simulink model "dynamics"  (R2016b)
settings: Solver=VariableStepAuto  StartTime=0.0  StopTime=10.0  RelTol=1e-3
values from neighbouring files (symbols this model uses):
  ModelInit_RPM = 557.1420    (= 557.142)    [Init.m]
  ModelParam_envGravityAcc = 9.8    [Init.m]
  ModelParam_motorCr = 1148*2    (= 2296)    [Init.m]
  ModelParam_motorJm = 0.0001287    [Init.m]
  ModelParam_motorT = 0.02    [Init.m]
  ModelParam_motorWb = -141.4    [Init.m]
  ModelParam_rotorCm = 1.779e-07    [Init.m]
  ModelParam_rotorCt = 1.105e-05    [Init.m]
  ModelParam_uavCd = 0.073    [Init.m]
  ModelParam_uavJ = [ModelParam_uavJxx,0,0;0,ModelParam_uavJyy,0;0,0,ModelParam_uavJzz]    [Init.m]
  ModelParam_uavMass = 1.4    [Init.m]
  ModelParam_uavR = 0.225    [Init.m]
libraries: aerolibutil x2, aerolibtransform2 x2
settings Model: Creator=Mr Wang  LastModifiedBy=Mr Wang

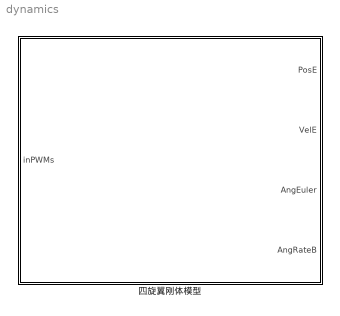
== system dynamics ==
  四旋翼刚体模型 : Subsystem
      mask Display: image('./icon/F450.png');

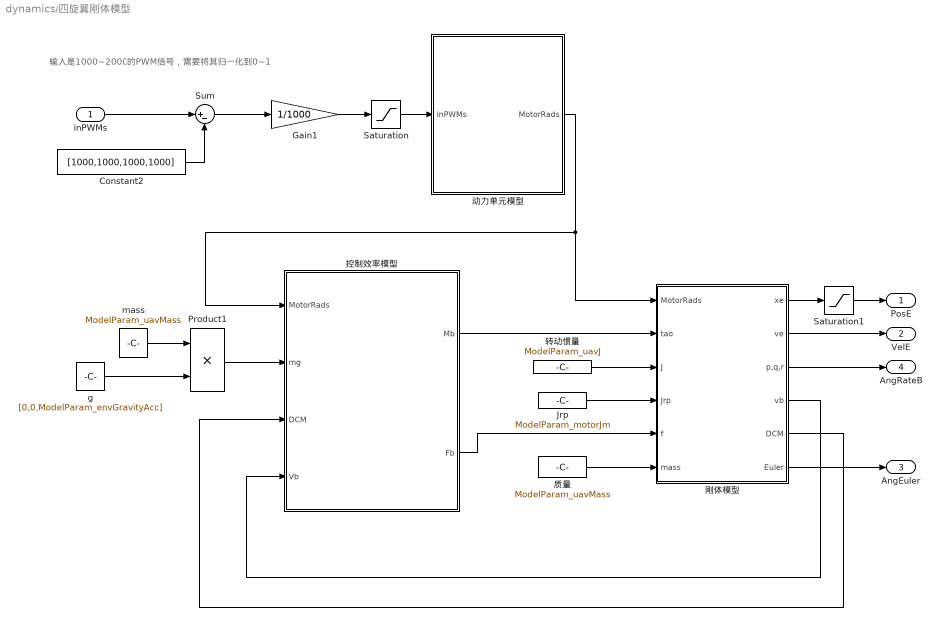
== system dynamics/四旋翼刚体模型 ==
  note: 输入是1000~2000的PWM信号，需要将其归一化到0~1
  inPWMs : Inport
  Constant2 : Constant  Value=[1000,1000,1000,1000]
  Gain1 : Gain  Gain=1/1000
  Jrp : Constant  Value=ModelParam_motorJm
  Product1 : Product
  Saturation : Saturate  UpperLimit=1  LowerLimit=0
  Saturation1 : Saturate  UpperLimit=[inf,inf,0]  LowerLimit=[-inf,-inf,-inf]
  Sum : Sum  Inputs=|+-
  g : Constant  Value=[0,0,ModelParam_envGravityAcc]
  mass : Constant  Value=ModelParam_uavMass
  刚体模型 : Subsystem
  动力单元模型 : Subsystem
  控制效率模型 : Subsystem
  质量 : Constant  Value=ModelParam_uavMass
  转动惯量 : Constant  Value=ModelParam_uavJ
  PosE : Outport
  VelE : Outport  Port=2
  AngEuler : Outport  Port=3
  AngRateB : Outport  Port=4
  wires:
  g/1 -> Product1/2
  Constant2/1 -> Sum/2
  控制效率模型/2(Fb) -> 刚体模型/5(f)
  inPWMs/1 -> Sum/1
  控制效率模型/1(Mb) -> 刚体模型/2(tao)
  刚体模型/6(Euler) -> AngEuler/1
  Saturation1/1 -> PosE/1
  刚体模型/4("vb ") -> 控制效率模型/4(Vb)
  Product1/1 -> 控制效率模型/2(mg)
  Sum/1 -> Gain1/1
  刚体模型/2(ve) -> VelE/1
  Gain1/1 -> Saturation/1
  转动惯量/1 -> 刚体模型/3(J)
  动力单元模型/1(MotorRads) -> 控制效率模型/1(MotorRads), 刚体模型/1(MotorRads)
  刚体模型/1("xe ") -> Saturation1/1
  刚体模型/5(DCM) -> 控制效率模型/3(DCM)
  mass/1 -> Product1/1
  质量/1 -> 刚体模型/6(mass)
  Jrp/1 -> 刚体模型/4(Jrp)
  刚体模型/3("p,q,r ") -> AngRateB/1
  Saturation/1 -> 动力单元模型/1(inPWMs)

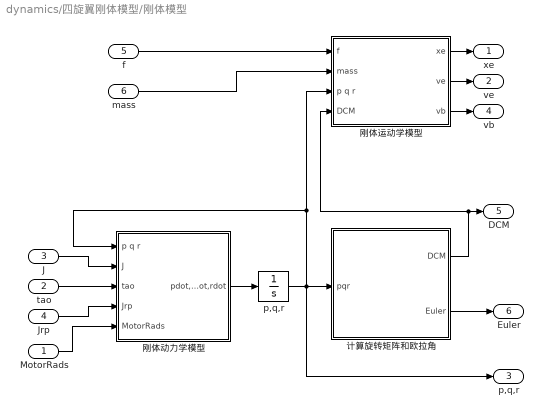
== system dynamics/四旋翼刚体模型/刚体模型 ==
  MotorRads : Inport
  tao : Inport  Port=2
  J : Inport  Port=3
  Jrp : Inport  Port=4
  f : Inport  Port=5
  mass : Inport  Port=6
  p,q,r : Integrator
  刚体动力学模型 : Subsystem
  刚体运动学模型 : Subsystem
  计算旋转矩阵和欧拉角 : Subsystem
  "xe " : Outport
  ve : Outport  Port=2
  "p,q,r " : Outport  Port=3
  "vb " : Outport  Port=4
  DCM : Outport  Port=5
  Euler : Outport  Port=6
  wires:
  J/1 -> 刚体动力学模型/2(J)
  tao/1 -> 刚体动力学模型/3(tao)
  Jrp/1 -> 刚体动力学模型/4(Jrp)
  MotorRads/1 -> 刚体动力学模型/5(MotorRads)
  刚体动力学模型/1(pdot,qdot,rdot) -> p,q,r/1
  计算旋转矩阵和欧拉角/1(DCM) -> DCM/1, 刚体运动学模型/4(DCM)
  计算旋转矩阵和欧拉角/2(Euler) -> Euler/1
  f/1 -> 刚体运动学模型/1(f)
  mass/1 -> 刚体运动学模型/2(mass)
  刚体运动学模型/1("xe ") -> "xe "/1
  刚体运动学模型/2(ve) -> ve/1
  p,q,r/1 -> 刚体运动学模型/3(p q r), 刚体动力学模型/1(p q r), "p,q,r "/1, 计算旋转矩阵和欧拉角/1(pqr)
  刚体运动学模型/3("vb ") -> "vb "/1

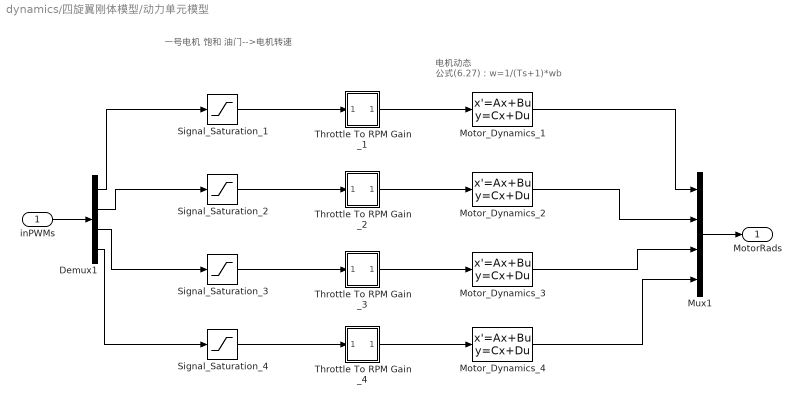
== system dynamics/四旋翼刚体模型/动力单元模型 ==
  note: 一号电机
      |
      |              饱和                             油门-->电机转速
  note: 电机动态
      | 公式(6.27)：w=1/(Ts+1)*wb
  inPWMs : Inport
  Demux1 : Demux
  Motor_Dynamics_{1..4} (4 alike) : StateSpace  A=-1/ModelParam_motorT  C=1/ModelParam_motorT  D=0  X0=ModelInit_RPM*ModelParam_motorT
  Mux1 : Mux
  Signal_Saturation_{1..4} (4 alike) : Saturate  UpperLimit=1  LowerLimit=0
  Throttle To RPM Gain _1 : Subsystem
  Throttle To RPM Gain _2 : Subsystem
  Throttle To RPM Gain _3 : Subsystem
  Throttle To RPM Gain _4 : Subsystem
  MotorRads : Outport
  wires:
  Demux1/1 -> Signal_Saturation_1/1
  Demux1/2 -> Signal_Saturation_2/1
  Demux1/3 -> Signal_Saturation_3/1
  Demux1/4 -> Signal_Saturation_4/1
  inPWMs/1 -> Demux1/1
  Throttle To RPM Gain _1/1(Out5) -> Motor_Dynamics_1/1
  Throttle To RPM Gain _2/1(Out5) -> Motor_Dynamics_2/1
  Throttle To RPM Gain _3/1(Out5) -> Motor_Dynamics_3/1
  Mux1/1 -> MotorRads/1
  Signal_Saturation_1/1 -> Throttle To RPM Gain _1/1(In5)
  Motor_Dynamics_1/1 -> Mux1/1
  Motor_Dynamics_2/1 -> Mux1/2
  Motor_Dynamics_3/1 -> Mux1/3
  Motor_Dynamics_4/1 -> Mux1/4
  Signal_Saturation_2/1 -> Throttle To RPM Gain _2/1(In5)
  Signal_Saturation_3/1 -> Throttle To RPM Gain _3/1(In5)
  Signal_Saturation_4/1 -> Throttle To RPM Gain _4/1(In5)
  Throttle To RPM Gain _4/1(Out5) -> Motor_Dynamics_4/1

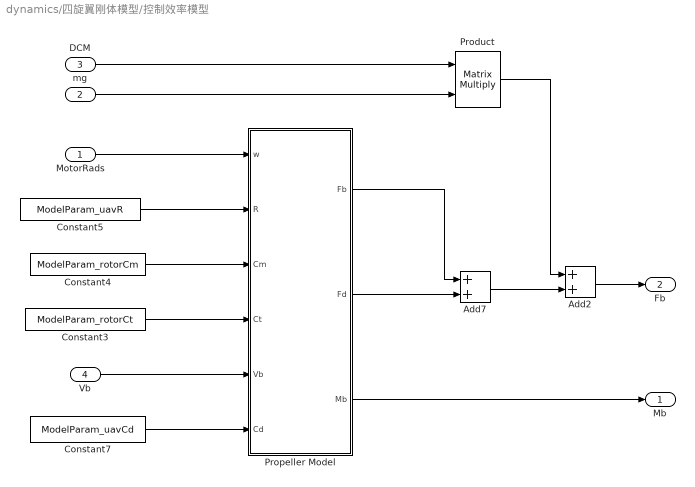
== system dynamics/四旋翼刚体模型/控制效率模型 ==
  MotorRads : Inport
  mg : Inport  Port=2
  DCM : Inport  Port=3
  Vb : Inport  Port=4
  Add2 : Sum
  Add7 : Sum
  Constant3 : Constant  Value=ModelParam_rotorCt
  Constant4 : Constant  Value=ModelParam_rotorCm
  Constant5 : Constant  Value=ModelParam_uavR
  Constant7 : Constant  Value=ModelParam_uavCd
  Product : Product  Multiplication=Matrix(*)
  Propeller Model : MATLAB Function  TreatAsAtomicUnit=on
  Mb : Outport
  Fb : Outport  Port=2
  wires:
  MotorRads/1 -> Propeller Model/1(w)
  Constant4/1 -> Propeller Model/3(Cm)
  Constant5/1 -> Propeller Model/2(R)
  Vb/1 -> Propeller Model/5(Vb)
  Constant7/1 -> Propeller Model/6(Cd)
  DCM/1 -> Product/1
  mg/1 -> Product/2
  Product/1 -> Add2/1
  Propeller Model/1(Fb) -> Add7/1
  Add7/1 -> Add2/2
  Propeller Model/2(Fd) -> Add7/2
  Constant3/1 -> Propeller Model/4(Ct)
  Add2/1 -> Fb/1
  Propeller Model/3(Mb) -> Mb/1

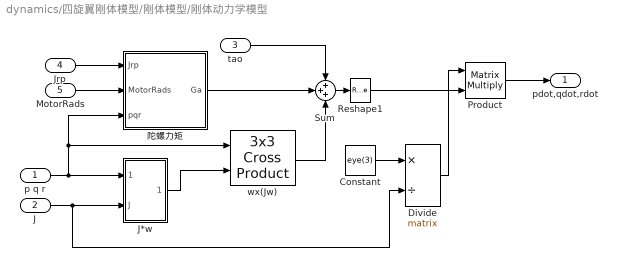
== system dynamics/四旋翼刚体模型/刚体模型/刚体动力学模型 ==
  p q r : Inport
  J : Inport  Port=2
  tao : Inport  Port=3
  Jrp : Inport  Port=4
  MotorRads : Inport  Port=5
  Constant : Constant  Value=eye(3)
  Divide : Product  Inputs=*/  Multiplication=Matrix(*)
  J*w : Subsystem
  Product : Product  Multiplication=Matrix(*)
  Reshape1 : Reshape  OutputDimensionality=Column vector (2-D)
  Sum : Sum  Inputs=3
  wx(Jw) : aerolibutil/3x3 Cross Product
  陀螺力矩 : MATLAB Function  TreatAsAtomicUnit=on
  pdot,qdot,rdot : Outport
  wires:
  wx(Jw)/1 -> Sum/3
  MotorRads/1 -> 陀螺力矩/2(MotorRads)
  Jrp/1 -> 陀螺力矩/1(Jrp)
  tao/1 -> Sum/1
  J*w/1("J*w ") -> wx(Jw)/2
  p q r/1 -> wx(Jw)/1, 陀螺力矩/3(pqr), J*w/1(p q r)
  J/1 -> J*w/2(J), Divide/2
  Sum/1 -> Reshape1/1
  Divide/1 -> Product/1
  陀螺力矩/1(Ga) -> Sum/2
  Constant/1 -> Divide/1
  Reshape1/1 -> Product/2
  Product/1 -> pdot,qdot,rdot/1

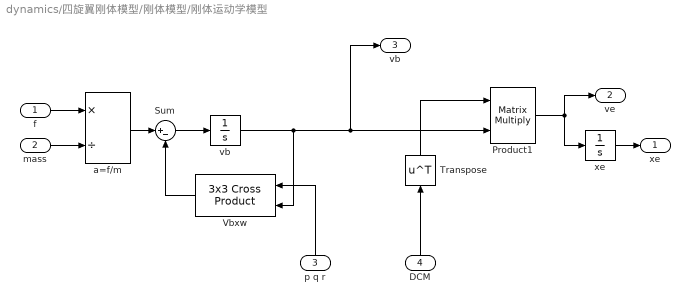
== system dynamics/四旋翼刚体模型/刚体模型/刚体运动学模型 ==
  f : Inport
  mass : Inport  Port=2
  p q r : Inport  Port=3
  DCM : Inport  Port=4
  Product1 : Product  Multiplication=Matrix(*)
  Sum : Sum  Inputs=|+-
  Transpose : Math  Operator=transpose  SaturateOnIntegerOverflow=on
  Vbxw : aerolibutil/3x3 Cross Product
  a=f/m : Product  Inputs=*/
  vb : Integrator
  xe : Integrator
  "xe " : Outport
  ve : Outport  Port=2
  "vb " : Outport  Port=3
  wires:
  DCM/1 -> Transpose/1
  p q r/1 -> Vbxw/1
  f/1 -> a=f/m/1
  Vbxw/1 -> Sum/2
  mass/1 -> a=f/m/2
  Transpose/1 -> Product1/1
  Product1/1 -> ve/1, xe/1
  xe/1 -> "xe "/1
  Sum/1 -> vb/1
  a=f/m/1 -> Sum/1
  vb/1 -> Vbxw/2, "vb "/1, Product1/2

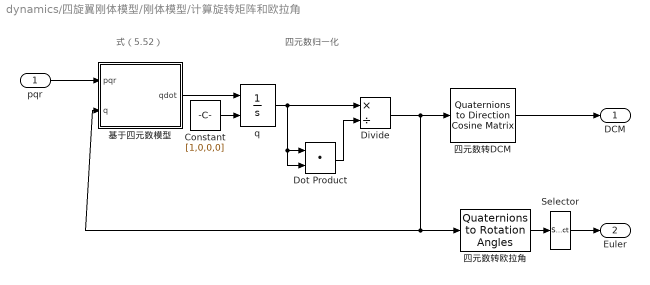
== system dynamics/四旋翼刚体模型/刚体模型/计算旋转矩阵和欧拉角 ==
  note: 四元数归一化
  note: 式（5.52）
  pqr : Inport
  Constant : Constant  Value=[1,0,0,0]
  Divide : Product  Inputs=*/
  Dot Product : DotProduct  InputSameDT=on  OutDataTypeStr=Inherit: Inherit via internal rule
  Selector : Selector  InputPortWidth=3  IndexOptions=Index vector (dialog)  Indices=[3 2 1]  OutputSizes=1
  q : Integrator  InitialConditionSource=external
  四元数转DCM : aerolibtransform2/Quaternions to  Direction Cosine Matrix
  四元数转欧拉角 : aerolibtransform2/Quaternions to Rotation Angles  rotationOrder=ZYX
  基于四元数模型 : MATLAB Function  TreatAsAtomicUnit=on
  DCM : Outport
  Euler : Outport  Port=2
  wires:
  Constant/1 -> q/2
  基于四元数模型/1(qdot) -> q/1
  q/1 -> Divide/1, Dot Product/2, Dot Product/1
  pqr/1 -> 基于四元数模型/1(pqr)
  四元数转DCM/1 -> DCM/1
  四元数转欧拉角/1 -> Selector/1
  Dot Product/1 -> Divide/2
  Divide/1 -> 四元数转欧拉角/1, 基于四元数模型/2(q), 四元数转DCM/1
  Selector/1 -> Euler/1

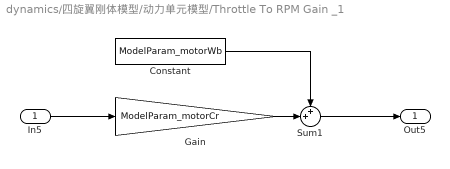
== system dynamics/四旋翼刚体模型/动力单元模型/Throttle To RPM Gain _1 ==
  In5 : Inport
  Constant : Constant  Value=ModelParam_motorWb
  Gain : Gain  Gain=ModelParam_motorCr
  Sum1 : Sum  Inputs=++|
  Out5 : Outport
  wires:
  Sum1/1 -> Out5/1
  In5/1 -> Gain/1
  Gain/1 -> Sum1/2
  Constant/1 -> Sum1/1

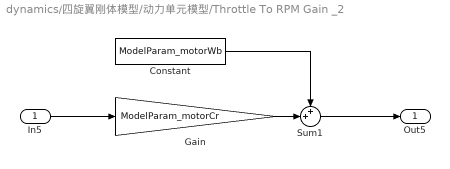
== system dynamics/四旋翼刚体模型/动力单元模型/Throttle To RPM Gain _2 ==
  In5 : Inport
  Constant : Constant  Value=ModelParam_motorWb
  Gain : Gain  Gain=ModelParam_motorCr
  Sum1 : Sum  Inputs=++|
  Out5 : Outport
  wires:
  Constant/1 -> Sum1/1
  Gain/1 -> Sum1/2
  In5/1 -> Gain/1
  Sum1/1 -> Out5/1

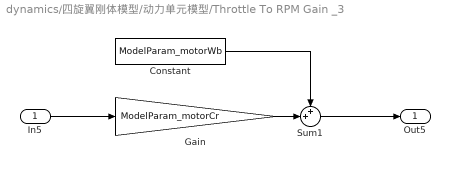
== system dynamics/四旋翼刚体模型/动力单元模型/Throttle To RPM Gain _3 ==
  In5 : Inport
  Constant : Constant  Value=ModelParam_motorWb
  Gain : Gain  Gain=ModelParam_motorCr
  Sum1 : Sum  Inputs=++|
  Out5 : Outport
  wires:
  Sum1/1 -> Out5/1
  In5/1 -> Gain/1
  Gain/1 -> Sum1/2
  Constant/1 -> Sum1/1

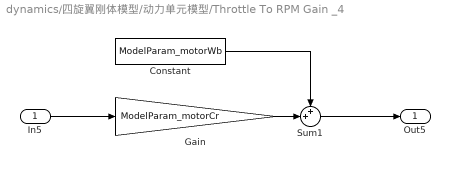
== system dynamics/四旋翼刚体模型/动力单元模型/Throttle To RPM Gain _4 ==
  In5 : Inport
  Constant : Constant  Value=ModelParam_motorWb
  Gain : Gain  Gain=ModelParam_motorCr
  Sum1 : Sum  Inputs=++|
  Out5 : Outport
  wires:
  Constant/1 -> Sum1/1
  Gain/1 -> Sum1/2
  In5/1 -> Gain/1
  Sum1/1 -> Out5/1

== system dynamics/四旋翼刚体模型/刚体模型/刚体动力学模型/J*w ==
  p q r : Inport
  J : Inport  Port=2
  J*w : Product  Multiplication=Matrix(*)
  "J*w " : Outport
  wires:
  p q r/1 -> J*w/2
  J/1 -> J*w/1
  J*w/1 -> "J*w "/1

== matlab function dynamics/四旋翼刚体模型/刚体模型/计算旋转矩阵和欧拉角/基于四元数模型 ==
  data: pqr input; qdot output; q input
function qdot = fcn(pqr,q)

qdot=0.5*[0,-pqr(1),-pqr(2),-pqr(3);pqr(1),0,pqr(3),-pqr(2);pqr(2),-pqr(3),0,pqr(1);pqr(3),pqr(2),-pqr(1),0]*q;

== matlab function dynamics/四旋翼刚体模型/刚体模型/刚体动力学模型/陀螺力矩 ==
  data: Jrp input; MotorRads input; pqr input; Ga output
function Ga = fcn(Jrp,MotorRads,pqr)
Ga=zeros(3,1);
Ga(1)=Jrp*pqr(2)*(-MotorRads(1)-MotorRads(2)+MotorRads(3)+MotorRads(4));
Ga(2)=Jrp*pqr(1)*( MotorRads(1)+MotorRads(2)-MotorRads(3)-MotorRads(4));

== matlab function dynamics/四旋翼刚体模型/控制效率模型/Propeller Model ==
  data: w input; R input; Fb output; Fd output; Mb output; Cm input; Ct input; Vb input; Cd input
function [Fb,Fd,Mb] = fcn(w,R,Cm,Ct,Vb,Cd)
 %%叉字型
 %3  1
 %2  4
 M_rctcm = [-sin(pi/4)*R*Ct,sin(pi/4)*R*Ct,sin(pi/4)*R*Ct,-sin(pi/4)*R*Ct;
            sin(pi/4)*R*Ct,-sin(pi/4)*R*Ct,sin(pi/4)*R*Ct,-sin(pi/4)*R*Ct;
            Cm,Cm,-Cm,-Cm];
 Mb = M_rctcm*(w.^2);%式(6.24),力矩
 
 Fb = [0; 0; -sum(Ct*(w.^2))]; %(6.23),螺旋桨拉力
 Fd = -Cd*Vb.*abs(Vb)*0.5;%空气阻力
end
